simulink model "PWM"  (R2020b)
settings: Solver=VariableStepAuto  StartTime=0.0  StopTime=10  RelTol=1e-3
libraries: dspswit3 x1, simulink x1
settings Model: Creator=ivans  LastModifiedBy=ivans

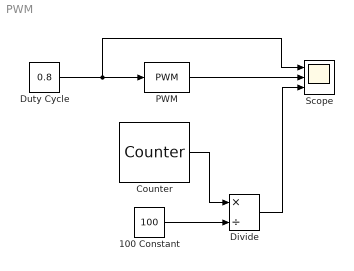
== system PWM ==
  100 Constant : Constant  Value=100
  Counter : dspswit3/Counter  Direction=Up  CountEvent=Free running  CounterSize=User defined  MaxCount=99  InitialCount=0  Output=Count  HitValue=32  ResetInput=off  SamplesPerFrame=1  Ts=0.01  CntDtype=uint8  HitDtype=Logical
  Divide : Product  Inputs=*/
  Duty Cycle : Constant  Value=0.8
  PWM : simulink/Discontinuities/PWM  DisableCoverage=on  Period=1  DisallowZeroDutyCycle=off  RunAtFixedTimeIntervals=on  SampleTime=0.1
  Scope : Scope  NumInputPorts=3
  wires:
  Duty Cycle/1 -> PWM/1, Scope/1
  PWM/1 -> Scope/2
  Counter/1 -> Divide/1
  Divide/1 -> Scope/3
  100 Constant/1 -> Divide/2
